simulink model "rhszero_discrete_2dof"  (R2014b)
settings: Solver=ode45  StartTime=0.0  StopTime=15  RelTol=1e-3
values from neighbouring files (symbols this model uses):
  aa = exp(-a*h)    [rhszero_variables.m]
  h = 0.05    [BLDC_partial2_fall18.m]    (also in abs_spring18.m = 0.2; active_suspension_ss.m = 0.00416985950901; active_suspension_ss_R.m = 0.00416985950901; active_suspension_ss_spring18.m = 0.004)
  r1 = s0s1r1(3)    [final_dummy.m]
  s0 = 2    [powerplant_dam_controllers.m]
  s1 = -1    [powerplant_dam_controllers.m]
  t0 = subs(Ac, z, 1) / subs(B, z, 1)    [abs_spring18.m]    (also in final_dummy.m = 3.67088607595; harddisk_discrete_design.m = 1/dcgain(Gcb); harddisk_discrete_design_2dof_example.m = 1/dcgain(Gcb))
libraries: simulink x1
settings Model: Creator=kjartan  LastModifiedBy=kjartan

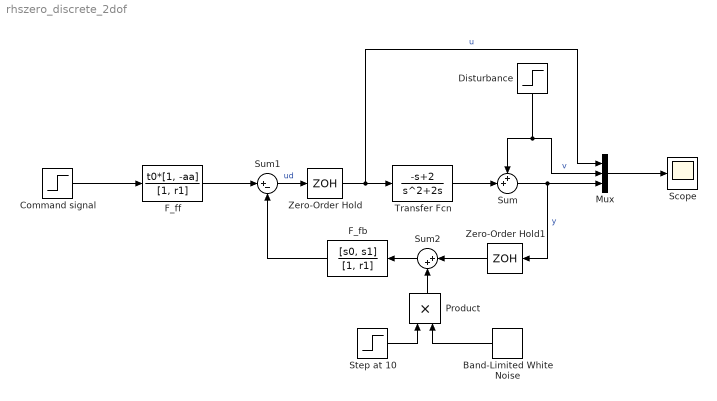
== system rhszero_discrete_2dof ==
  Band-Limited White Noise : simulink/Sources/Band-Limited White Noise  Cov=[0.02^2]  Ts=h  seed=[23341]
  Command signal : Step  Time=0  SampleTime=0
  Disturbance : Step  Time=5  SampleTime=0
  F_fb : DiscreteTransferFcn  Numerator=[s0, s1]  Denominator=[1, r1]  SampleTime=h
  F_ff : DiscreteTransferFcn  Numerator=t0*[1, -aa]  Denominator=[1, r1]  SampleTime=h
  Mux : Mux  Inputs=3
  Product : Product
  Scope : Scope
      settings: ShowLegends=on
  Step at 10 : Step  Time=10  SampleTime=0
  Sum : Sum  Inputs=++|
  Sum1 : Sum  Inputs=|+-
  Sum2 : Sum  Inputs=|++
  Transfer Fcn : TransferFcn  Numerator=[-1, 2]  Denominator=[1, 2, 0]
  Zero-Order Hold : ZeroOrderHold  SampleTime=h
  Zero-Order Hold1 : ZeroOrderHold  SampleTime=h
  wires:
  Sum/1 -> Zero-Order Hold1/1, Mux/3  "y"
  Transfer Fcn/1 -> Sum/2
  Mux/1 -> Scope/1
  Command signal/1 -> F_ff/1
  Disturbance/1 -> Sum/1, Mux/2  "v"
  Sum1/1 -> Zero-Order Hold/1  "ud"
  F_fb/1 -> Sum1/2
  F_ff/1 -> Sum1/1
  Zero-Order Hold/1 -> Transfer Fcn/1, Mux/1  "u"
  Step at 10/1 -> Product/1
  Band-Limited White Noise/1 -> Product/2
  Product/1 -> Sum2/2
  Zero-Order Hold1/1 -> Sum2/1
  Sum2/1 -> F_fb/1
